simulink library "parallel_protection_lib"  (R2018b)
settings: Solver=VariableStepAuto  StartTime=0.0  StopTime=10.0  RelTol=1e-3
settings Model: Creator=taylorreynolds  LastModifiedBy=taylorreynolds

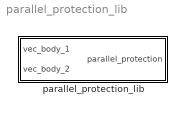
== system parallel_protection_lib ==
  parallel_protection_lib : Subsystem  mask{min_angle_deg=1.5}
      mask prompts: min_angle_deg "Angle [deg]"
      mask TypeOptions min_angle_deg: min_angle_deg/Value
      mask DialogControl DescTextVar Prompt: Enter the minimum angle difference between vectors to be considered "parallel"

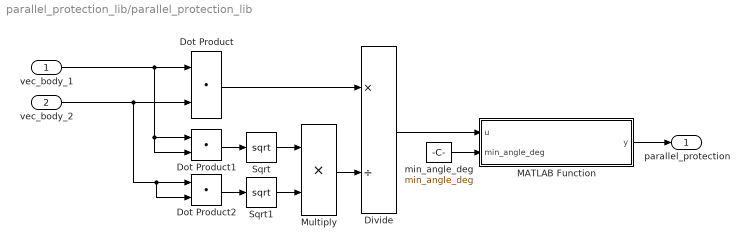
== system parallel_protection_lib/parallel_protection_lib ==
  vec_body_1 : Inport
  vec_body_2 : Inport  Port=2
  Divide : Product  Inputs=*/
  Dot Product : DotProduct  InputSameDT=on  OutDataTypeStr=Inherit: Inherit via internal rule
  Dot Product1 : DotProduct  InputSameDT=on  OutDataTypeStr=Inherit: Inherit via internal rule
  Dot Product2 : DotProduct  InputSameDT=on  OutDataTypeStr=Inherit: Inherit via internal rule
  MATLAB Function : MATLAB Function  TreatAsAtomicUnit=on
  Multiply : Product
  Sqrt : Sqrt  SaturateOnIntegerOverflow=on
  Sqrt1 : Sqrt  SaturateOnIntegerOverflow=on
  min_angle_deg : Constant  Value=min_angle_deg
  parallel_protection : Outport
  wires:
  vec_body_1/1 -> Dot Product1/1, Dot Product1/2, Dot Product/1
  Dot Product2/1 -> Sqrt1/1
  Sqrt/1 -> Multiply/1
  Multiply/1 -> Divide/2
  Dot Product/1 -> Divide/1
  Sqrt1/1 -> Multiply/2
  Divide/1 -> MATLAB Function/1(u)
  Dot Product1/1 -> Sqrt/1
  vec_body_2/1 -> Dot Product2/2, Dot Product2/1, Dot Product/2
  MATLAB Function/1(y) -> parallel_protection/1
  min_angle_deg/1 -> MATLAB Function/2(min_angle_deg)

== matlab function parallel_protection_lib/MATLAB Function ==
  data: u input size=1; y output boolean size=1; min_angle_deg input size=1
function y = check_angle(u,min_angle_deg)
%#codegen
y = false;
if abs(u) <= cosd(min_angle_deg)
    y = true;
else
end
